simulink model "Gamboa_Edrian_Simulink_No6"  (R2023b)
settings: Solver=VariableStepAuto  StartTime=0.0  StopTime=20  RelTol=1e-3
values from neighbouring files (symbols this model uses):
  G_den = [b c d]    [DeRamos_MacGleen_MATLAB_No1.m]    (also in DeRamos_MacGleen_MATLAB_No2.m; Dimapasoc_Cassius_MATLAB_No3.m; Dimapasoc_Cassius_MATLAB_No4.m = [b c]; Gamboa_Edrian_MATLAB_No5.m = [h i j k l m n o])
  G_num = [a]    [DeRamos_MacGleen_MATLAB_No1.m]    (also in DeRamos_MacGleen_MATLAB_No2.m; Dimapasoc_Cassius_MATLAB_No3.m; Dimapasoc_Cassius_MATLAB_No4.m; Gamboa_Edrian_MATLAB_No5.m = [a b c d e f g])
settings Model: Creator=Edrian Gamboa  LastModifiedBy=Edrian Gamboa

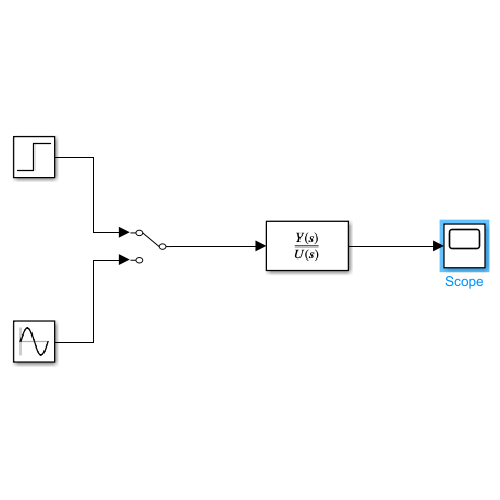
[thumbnail: Simulink's stored preview of the top-level diagram]
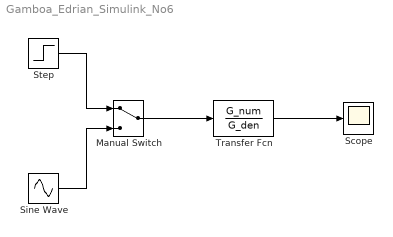
== system Gamboa_Edrian_Simulink_No6 ==
  Manual Switch : ManualSwitch
  Scope : Scope
  Sine Wave : Sin  SampleTime=0
  Step : Step  Time=0.1  SampleTime=0
  Transfer Fcn : TransferFcn  Numerator=G_num  Denominator=G_den
  wires:
  Step/1 -> Manual Switch/1
  Sine Wave/1 -> Manual Switch/2
  Manual Switch/1 -> Transfer Fcn/1
  Transfer Fcn/1 -> Scope/1
